simulink model "PositionValidation"  (R2022b)
settings: Solver=VariableStepAuto  StartTime=0.0  StopTime=10.0  RelTol=1e-3
StopFcn:
  | inverse_kinematics_func
settings Model: Creator=DELL  LastModifiedBy=DELL

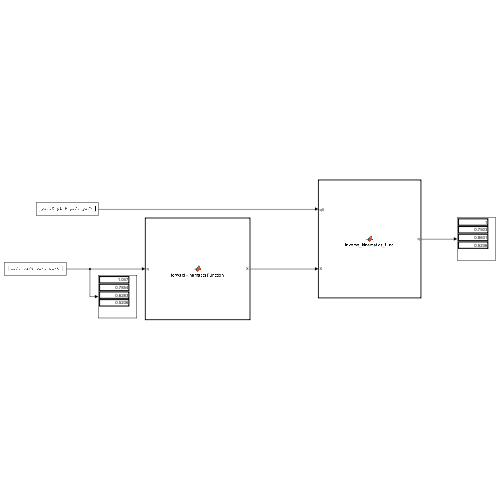
[thumbnail: Simulink's stored preview of the top-level diagram]
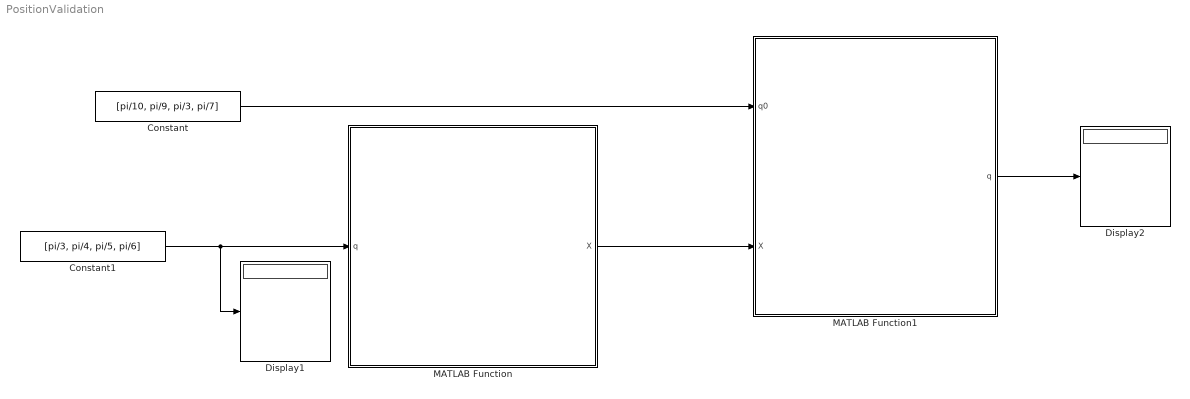
== system PositionValidation ==
  Constant : Constant  Value=[pi/10, pi/9, pi/3, pi/7]
  Constant1 : Constant  Value=[pi/3, pi/4, pi/5, pi/6]
  Display1 : Display
  Display2 : Display
  MATLAB Function : MATLAB Function  TreatAsAtomicUnit=on
  MATLAB Function1 : MATLAB Function  TreatAsAtomicUnit=on
  wires:
  MATLAB Function1/1(q) -> Display2/1
  Constant1/1 -> Display1/1, MATLAB Function/1(q)
  Constant/1 -> MATLAB Function1/1(q0)
  MATLAB Function/1(X) -> MATLAB Function1/2(X)

== matlab function PositionValidation/MATLAB Function1 ==
  data: q output; q0 input; X input
function q = inverse_kinematics_func(q0, X)
q = [0; 0; 0; 0];
n = 0;

while n < 1000
    
    q1 = q0(1);
    q2 = q0(2);
    q3 = q0(3);
    q4 = q0(4);

    partialFpartialQ = [150*sin(q2)*sin(q1 - pi/2)*sin(q4 - pi/2) - 150*cos(q4 - pi/2)*(cos(q1 - pi/2)*sin(q3 - pi/2) + cos(q2)*cos(q3 - pi/2)*sin(q1 - pi/2)) - 185*sin(q2)*sin(q1 - pi/2), 185*cos(q2)*cos(q1 - pi/2) - 150*cos(q2)*cos(q1 - pi/2)*sin(q4 - pi/2) - 150*cos(q1 - pi/2)*cos(q3 - pi/2)*cos(q4 - pi/2)*sin(q2), -150*cos(q4 - pi/2)*(cos(q3 - pi/2)*sin(q1 - pi/2) + cos(q2)*cos(q1 - pi/2)*sin(q3 - pi/2)),   150*sin(q4 - pi/2)*(sin(q1 - pi/2)*sin(q3 - pi/2) - cos(q2)*cos(q1 - pi/2)*cos(q3 - pi/2)) - 150*cos(q1 - pi/2)*cos(q4 - pi/2)*sin(q2);
    185*cos(q1 - pi/2)*sin(q2) - 150*cos(q4 - pi/2)*(sin(q1 - pi/2)*sin(q3 - pi/2) - cos(q2)*cos(q1 - pi/2)*cos(q3 - pi/2)) - 150*cos(q1 - pi/2)*sin(q2)*sin(q4 - pi/2), 185*cos(q2)*sin(q1 - pi/2) - 150*cos(q2)*sin(q1 - pi/2)*sin(q4 - pi/2) - 150*cos(q3 - pi/2)*cos(q4 - pi/2)*sin(q2)*sin(q1 - pi/2),  150*cos(q4 - pi/2)*(cos(q1 - pi/2)*cos(q3 - pi/2) - cos(q2)*sin(q1 - pi/2)*sin(q3 - pi/2)), - 150*sin(q4 - pi/2)*(cos(q1 - pi/2)*sin(q3 - pi/2) + cos(q2)*cos(q3 - pi/2)*sin(q1 - pi/2)) - 150*cos(q4 - pi/2)*sin(q2)*sin(q1 - pi/2);
    0,                                              150*sin(q2)*sin(q4 - pi/2) - 185*sin(q2) - 150*cos(q2)*cos(q3 - pi/2)*cos(q4 - pi/2),                                                   150*cos(q4 - pi/2)*sin(q2)*sin(q3 - pi/2),                                                                   150*cos(q3 - pi/2)*sin(q2)*sin(q4 - pi/2) - 150*cos(q2)*cos(q4 - pi/2)];

xee = 185*cos(q1 - pi/2)*sin(q2)...
    - 150*cos(q4 - pi/2)*(sin(q1 - pi/2)*sin(q3 - pi/2)...
    - cos(q2)*cos(q1 - pi/2)*cos(q3 - pi/2))...
    - 150*cos(q1 - pi/2)*sin(q2)*sin(q4 - pi/2);

yee = 185*sin(q2)*sin(q1 - pi/2)...
    + 150*cos(q4 - pi/2)*(cos(q1 - pi/2)*sin(q3 - pi/2)...
    + cos(q2)*cos(q3 - pi/2)*sin(q1 - pi/2))...
    - 150*sin(q2)*sin(q1 - pi/2)*sin(q4 - pi/2);

zee = 185*cos(q2) - 150*cos(q2)*sin(q4 - pi/2)...
    - 150*cos(q3 - pi/2)*cos(q4 - pi/2)*sin(q2) + 27;


    Jinv = pinv(partialFpartialQ);
    q = q0 - Jinv * [xee - X(1); yee - X(2); zee - X(3)];
    q(1) = wrapTo2Pi(q(1));
    q(2) = wrapTo2Pi(q(2));
    q(3) = wrapTo2Pi(q(3));
    q(4) = wrapTo2Pi(q(4));
    q0 = q;
    n = n + 1;
end
end

== matlab function PositionValidation/MATLAB Function ==
  data: q input; X output
function X =  forwardKinematicsFunction(q)

q1 = q(1);
q2 = q(2);
q3 = q(3);
q4 = q(4);

xee = 185*cos(q1 - pi/2)*sin(q2)...
    - 150*cos(q4 - pi/2)*(sin(q1 - pi/2)*sin(q3 - pi/2)...
    - cos(q2)*cos(q1 - pi/2)*cos(q3 - pi/2))...
    - 150*cos(q1 - pi/2)*sin(q2)*sin(q4 - pi/2);
 
yee = 185*sin(q2)*sin(q1 - pi/2)...
    + 150*cos(q4 - pi/2)*(cos(q1 - pi/2)*sin(q3 - pi/2)...
    + cos(q2)*cos(q3 - pi/2)*sin(q1 - pi/2))...
    - 150*sin(q2)*sin(q1 - pi/2)*sin(q4 - pi/2);
 
zee = 185*cos(q2) - 150*cos(q2)*sin(q4 - pi/2)...
    - 150*cos(q3 - pi/2)*cos(q4 - pi/2)*sin(q2) + 27;
X = [xee; yee; zee];

 
end
